simulink model "srp_test"  (R2023b)
settings: Solver=VariableStepAuto  StartTime=0.0  StopTime=10.0  RelTol=1e-3
undefined symbols (not defined in the file): Environment
libraries: dyn_lib x3
settings Model: DataDictionary=Scenario.sldd  Creator=brent  LastModifiedBy=brent

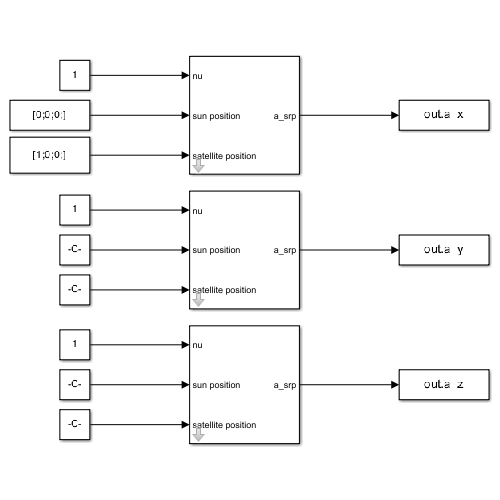
[thumbnail: Simulink's stored preview of the top-level diagram]
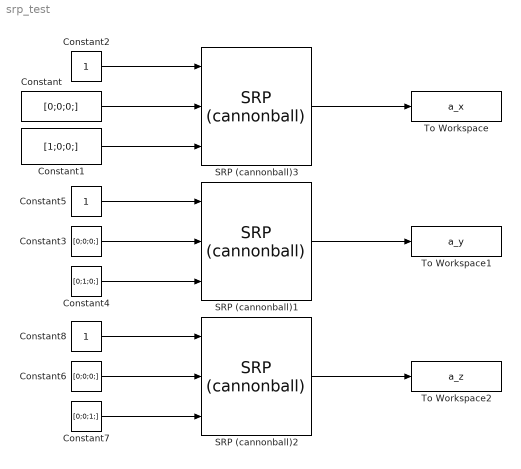
== system srp_test ==
  Constant : Constant  Value=[0;0;0;]
  Constant1 : Constant  Value=[1;0;0;]
  Constant2 : Constant
  Constant3 : Constant  Value=[0;0;0;]
  Constant4 : Constant  Value=[0;1;0;]
  Constant5 : Constant
  Constant6 : Constant  Value=[0;0;0;]
  Constant7 : Constant  Value=[0;0;1;]
  Constant8 : Constant
  SRP (cannonball)1 : dyn_lib/SRP (cannonball)  C_R=1  A_sc=1  m=1  AU=Environment.AU.value  P=Environment.Sun.P.value
      settings: SourceProductName=Dynamics library
  SRP (cannonball)2 : dyn_lib/SRP (cannonball)  C_R=1  A_sc=1  m=1  AU=Environment.AU.value  P=Environment.Sun.P.value
      settings: SourceProductName=Dynamics library
  SRP (cannonball)3 : dyn_lib/SRP (cannonball)  C_R=1  A_sc=1  m=1  AU=Environment.AU.value  P=Environment.Sun.P.value
      settings: SourceProductName=Dynamics library
  To Workspace : ToWorkspace  VariableName=a_x  SampleTime=-1
      settings: Save2DSignal=2-D array (concatenate along first dimension)
  To Workspace1 : ToWorkspace  VariableName=a_y  SampleTime=-1
      settings: Save2DSignal=2-D array (concatenate along first dimension)
  To Workspace2 : ToWorkspace  VariableName=a_z  SampleTime=-1
      settings: Save2DSignal=2-D array (concatenate along first dimension)
  wires:
  Constant/1 -> SRP (cannonball)3/2
  Constant1/1 -> SRP (cannonball)3/3
  Constant2/1 -> SRP (cannonball)3/1
  SRP (cannonball)3/1 -> To Workspace/1
  SRP (cannonball)1/1 -> To Workspace1/1
  Constant3/1 -> SRP (cannonball)1/2
  Constant4/1 -> SRP (cannonball)1/3
  Constant5/1 -> SRP (cannonball)1/1
  SRP (cannonball)2/1 -> To Workspace2/1
  Constant6/1 -> SRP (cannonball)2/2
  Constant7/1 -> SRP (cannonball)2/3
  Constant8/1 -> SRP (cannonball)2/1
